simulink model "shock_motion"  (R2022b)
settings: Solver=ode45  StartTime=0.0  StopTime=15  FixedStep=.1  RelTol=1e-3  EnableMultiTasking=on
PreLoadFcn:
  | % Parameters
  | M = 1;  % Mass of vehicle [kg]
  | Cd = 1; % Damping constant [N/(m/s)]
  | Cs = 2; % Spring constant [N/m]
settings Model: Creator=jrivitus  LastModifiedBy=bensweet
settings SolverCC: AlgebraicLoopSolver=TrustRegion
settings DataIOCC: LimitDataPoints=on  SaveFormat=Array  ReturnWorkspaceOutputs=off
settings OptimizationCC: ExpressionDepthLimit=2147483647  InitFltsAndDblsToZero=on  LifeSpan=inf
settings DebuggingCC: UnconnectedInputMsg=warning  UnconnectedOutputMsg=warning  UnconnectedLineMsg=warning  PregeneratedLibrarySubsystemCodeDiagnostic=none  SFMachineParentedDataDiag=warning
settings HardwareCC: ProdBitPerPointer=32  ProdBitPerSizeT=32  ProdBitPerPtrDiffT=32  ProdLargestAtomicFloat=None  ProdIntDivRoundTo=Undefined  ProdEndianess=Unspecified  ProdWordSize=32  ProdHWDeviceType=32-bit Generic
settings ModelReferenceCC: EnableRefExpFcnMdlSchedulingChecks=on  PropagateSignalLabelsOutOfModel=off
settings SFSimCC: SimUseLocalCustomCode=off
settings RTWCC: RTWUseLocalCustomCode=off  DLArmComputeVersion=19.05
settings CodeAppCC: StateflowObjectComments=on
settings GRTTargetCC: TargetFcnLib=ansi_tfl_tmw.mat  TargetLangStandard=C89/C90 (ANSI)  CombineOutputUpdateFcns=off  GRTInterface=on
settings ConfigComp: CovMetricSettings=dw  CovSaveCumulativeToWorkspaceVar=on  CovSaveSingleToWorkspaceVar=on  CovExternalEMLEnable=off  CovSFcnEnable=off

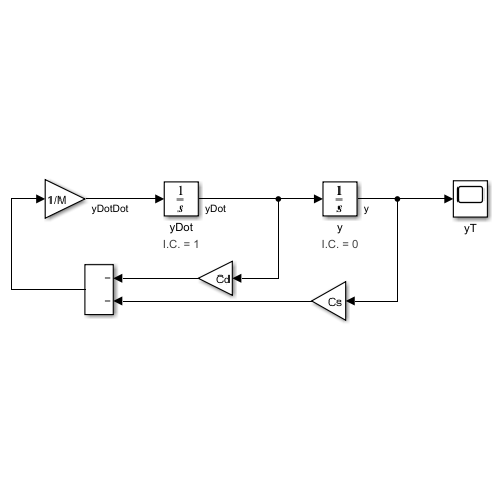
[thumbnail: Simulink's stored preview of the top-level diagram]
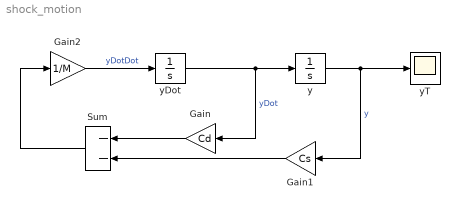
== system shock_motion ==
  Gain : Gain  Gain=Cd
  Gain1 : Gain  Gain=Cs
  Gain2 : Gain  Gain=1/M
  Sum : Sum  Inputs=--
  y : Integrator
      settings: AttributesFormatString=I.C. = %<InitialCondition>
  yDot : Integrator  InitialCondition=1
      settings: AttributesFormatString=I.C. = %<InitialCondition>
  yT : Scope
  wires:
  y/1 -> Gain1/1, yT/1  "y"
  yDot/1 -> y/1, Gain/1  "yDot"
  Sum/1 -> Gain2/1
  Gain/1 -> Sum/1
  Gain1/1 -> Sum/2
  Gain2/1 -> yDot/1  "yDotDot"
